simulink model "Simu_Workclass1"  (R2016a)
settings: Solver=VariableStepAuto  StartTime=0.0  StopTime=10.0  RelTol=1e-3
libraries: simulink x2
settings Model: Creator=Pection  LastModifiedBy=Pection

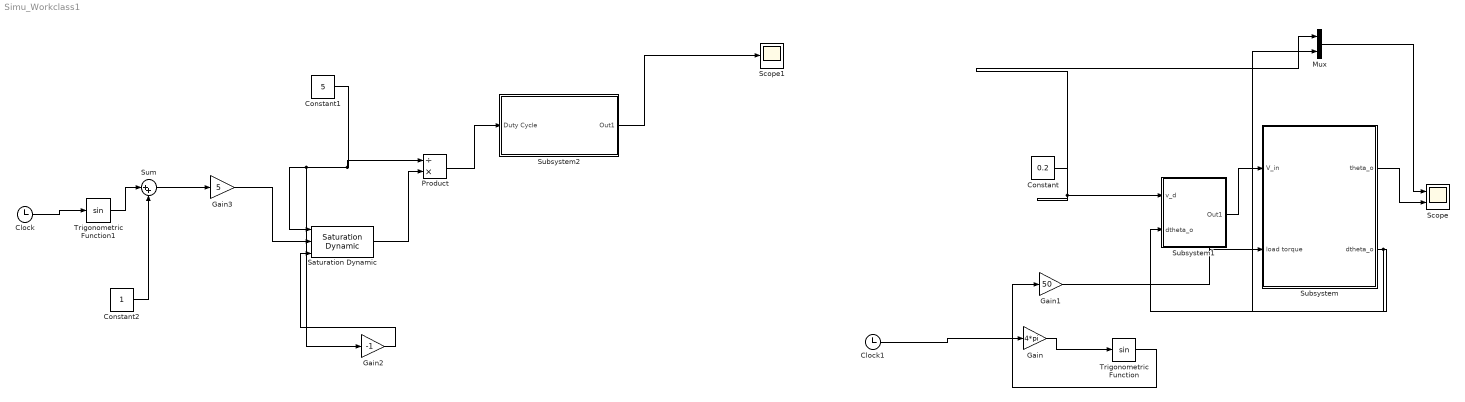
== system Simu_Workclass1 ==
  Clock : Clock
  Clock1 : Clock
  Constant : Constant  Value=0.2
  Constant1 : Constant  Value=5
  Constant2 : Constant
  Gain : Gain  Gain=4*pi
  Gain1 : Gain  Gain=50
  Gain2 : Gain  Gain=-1
  Gain3 : Gain  Gain=5
  Mux : Mux  Inputs=2
  Product : Product  Inputs=/*
  Saturation Dynamic : simulink/Discontinuities/Saturation Dynamic  OutMin=[]  OutMax=[]  OutDataTypeStr=Inherit: Same as second input  OutDataType=fixdt(1, 16)  OutScaling=2^-10  DoSatur=off
  Scope : Scope  NumInputPorts=2
  Scope1 : Scope
  Subsystem : Subsystem  mask(Dc_motor){j_m=2, B_m=0.1, rg=20, L=0.1, K_b=1, K_m=10, R=10}
      mask prompts: j_m "Motor Inertial"; B_m "Damp"; rg "Gear Ratio"; L "Inductor"; K_b "Kb"; K_m "Km"; R "Resistance"
      mask help: Homework
  Subsystem1 : Subsystem  mask{K_i=70, K_p=150}
      mask prompts: K_i "Ki"; K_p "Kp"
  Subsystem2 : Subsystem  mask{f=20}
      mask prompts: f "fre"
  Sum : Sum  Inputs=|++
  Trigonometric Function : Trigonometry
  Trigonometric Function1 : Trigonometry
  wires:
  Subsystem1/1(Out1) -> Subsystem/1(V_in)
  Constant/1 -> Mux/1, Subsystem1/1(v_d)
  Subsystem/2(dtheta_o) -> Mux/2, Subsystem1/2("dtheta_o ")
  Mux/1 -> Scope/1
  Subsystem/1("theta_o ") -> Scope/2
  Gain1/1 -> Subsystem/2("load torque ")
  Clock1/1 -> Gain/1
  Trigonometric Function/1 -> Gain1/1
  Gain/1 -> Trigonometric Function/1
  Subsystem2/1(Out1) -> Scope1/1
  Gain2/1 -> Saturation Dynamic/3
  Saturation Dynamic/1 -> Product/2
  Product/1 -> Subsystem2/1(Duty Cycle)
  Clock/1 -> Trigonometric Function1/1
  Trigonometric Function1/1 -> Sum/1
  Constant2/1 -> Sum/2
  Sum/1 -> Gain3/1
  Gain3/1 -> Saturation Dynamic/2
  Constant1/1 -> Product/1, Saturation Dynamic/1, Gain2/1

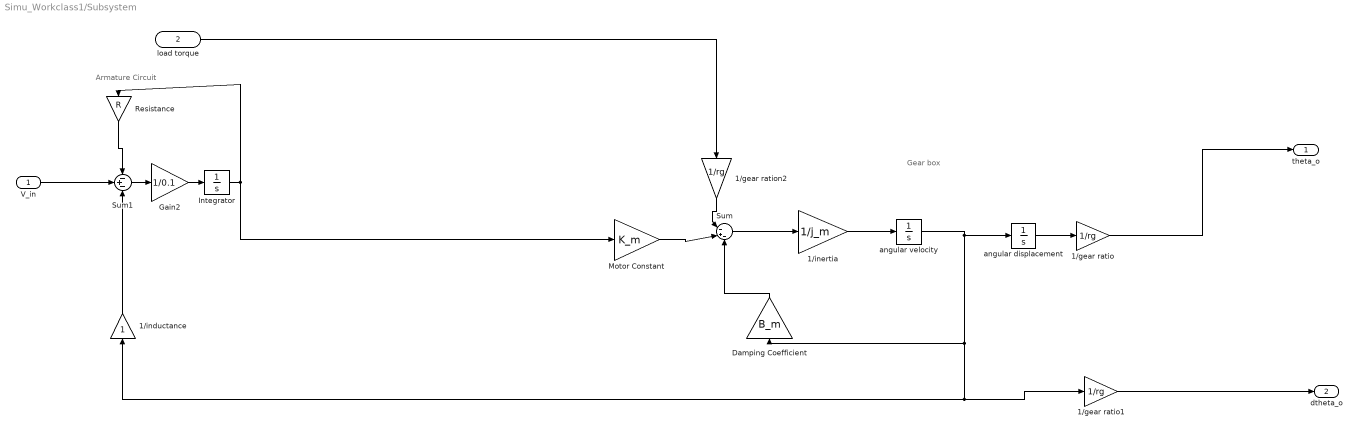
== system Simu_Workclass1/Subsystem ==
  note: Gear box
  note: Armature Circuit
  V_in : Inport
  "load torque " : Inport  Port=2
  1/gear ratio : Gain  Gain=1/rg
  1/gear ratio1 : Gain  Gain=1/rg
  1/gear ration2 : Gain  Gain=1/rg
  1/inductance : Gain
  "1/inertia " : Gain  Gain=1/j_m
  Damping Coefficient : Gain  Gain=B_m
  Gain2 : Gain  Gain=1/0.1
  Integrator : Integrator
  Motor Constant : Gain  Gain=K_m
  "Resistance " : Gain  Gain=R
  Sum : Sum  Inputs=|-+-
  Sum1 : Sum  Inputs=-+-
  angular displacement : Integrator
  "angular velocity " : Integrator
  "theta_o " : Outport
  dtheta_o : Outport  Port=2
  wires:
  angular displacement/1 -> 1/gear ratio/1
  Sum/1 -> "1/inertia "/1
  "Resistance "/1 -> Sum1/1
  V_in/1 -> Sum1/2
  1/inductance/1 -> Sum1/3
  1/gear ratio/1 -> "theta_o "/1
  Gain2/1 -> Integrator/1
  Sum1/1 -> Gain2/1
  1/gear ratio1/1 -> dtheta_o/1
  "angular velocity "/1 -> 1/inductance/1, 1/gear ratio1/1, Damping Coefficient/1, angular displacement/1
  1/gear ration2/1 -> Sum/1
  "load torque "/1 -> 1/gear ration2/1
  "1/inertia "/1 -> "angular velocity "/1
  Damping Coefficient/1 -> Sum/3
  Motor Constant/1 -> Sum/2
  Integrator/1 -> Motor Constant/1, "Resistance "/1

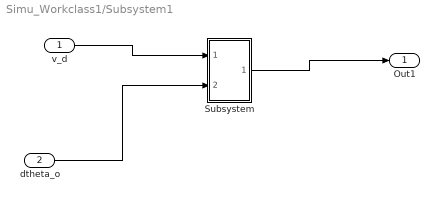
== system Simu_Workclass1/Subsystem1 ==
  v_d : Inport
  "dtheta_o " : Inport  Port=2
  Subsystem : Subsystem
  Out1 : Outport
  wires:
  v_d/1 -> Subsystem/1(v_d)
  "dtheta_o "/1 -> Subsystem/2("dtheta_o ")
  Subsystem/1(Out1) -> Out1/1

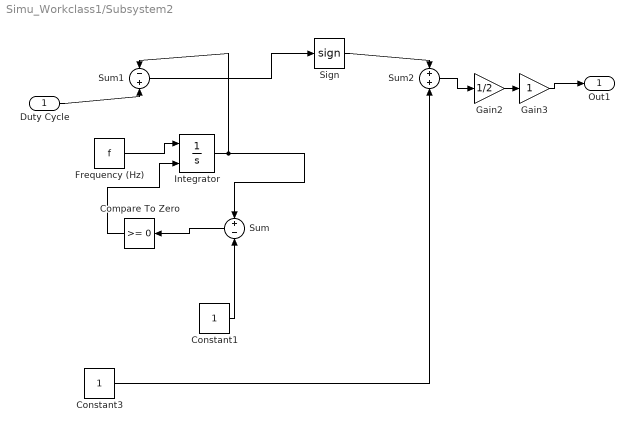
== system Simu_Workclass1/Subsystem2 ==
  Duty Cycle : Inport
  Compare To Zero : simulink/Logic and Bit Operations/Compare To Zero  relop=>=  OutDataTypeStr=boolean
  Constant1 : Constant
  Constant3 : Constant
  Frequency (Hz) : Constant  Value=f
  Gain2 : Gain  Gain=1/2
  Gain3 : Gain
  Integrator : Integrator  ExternalReset=rising
  Sign : Signum
  Sum : Sum  Inputs=+-
  Sum1 : Sum  Inputs=-+
  Sum2 : Sum
  Out1 : Outport
  wires:
  Constant1/1 -> Sum/2
  Integrator/1 -> Sum/1, Sum1/1
  Frequency (Hz)/1 -> Integrator/1
  Sum1/1 -> Sign/1
  Sign/1 -> Sum2/1
  Sum/1 -> Compare To Zero/1
  Compare To Zero/1 -> Integrator/2
  Constant3/1 -> Sum2/2
  Duty Cycle/1 -> Sum1/2
  Gain3/1 -> Out1/1
  Sum2/1 -> Gain2/1
  Gain2/1 -> Gain3/1

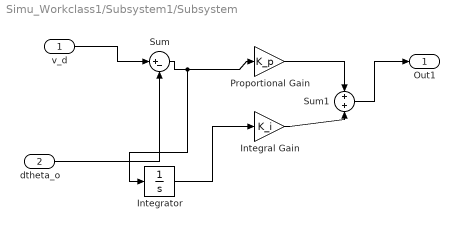
== system Simu_Workclass1/Subsystem1/Subsystem ==
  v_d : Inport
  "dtheta_o " : Inport  Port=2
  Integral Gain : Gain  Gain=K_i
  Integrator : Integrator
  "Proportional Gain " : Gain  Gain=K_p
  Sum : Sum  Inputs=|+-
  Sum1 : Sum
  Out1 : Outport
  wires:
  Integrator/1 -> Integral Gain/1
  v_d/1 -> Sum/1
  Sum/1 -> Integrator/1, "Proportional Gain "/1
  "Proportional Gain "/1 -> Sum1/1
  Sum1/1 -> Out1/1
  Integral Gain/1 -> Sum1/2
  "dtheta_o "/1 -> Sum/2
